simulink model "Model_HVAC_final_Lidia Garcia"  (R2020b)
settings: Solver=VariableStepAuto  StartTime=0.0  StopTime=8760  RelTol=1e-3
undefined symbols (not defined in the file or in its folder): sigbuilder_block
settings Model: Creator=HP  LastModifiedBy=HP
settings SolverCC: ZeroCrossAlgorithm=Adaptive
settings DebuggingCC: IgnoredZcDiagnostic=none  ArithmeticOperatorsInVariantConditions=warning
settings SFSimCC: CustomCodeUndefinedFunction=UseInterfaceOnly

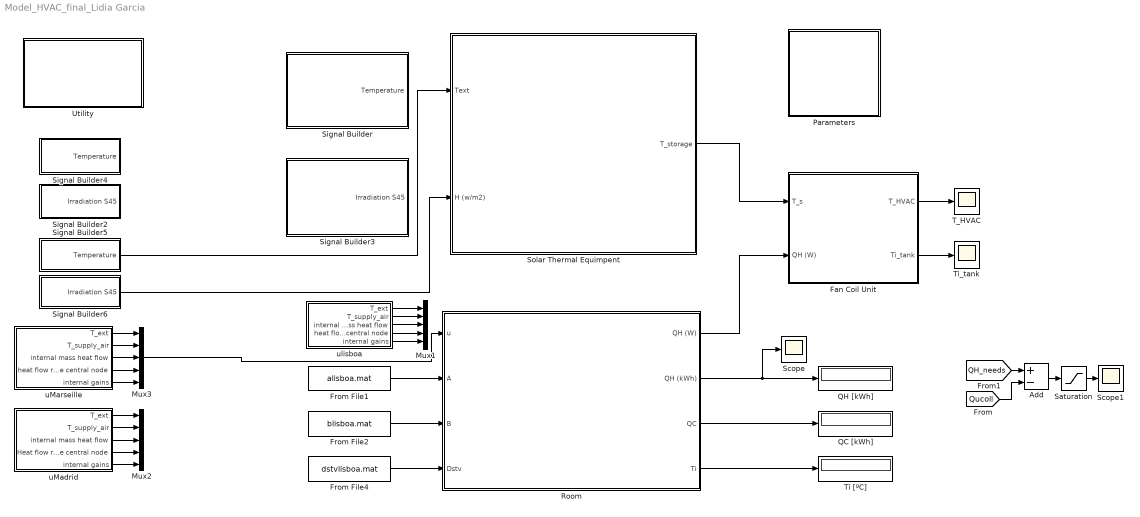
== system Model_HVAC_final_Lidia Garcia ==
  Add : Sum  Inputs=+-
  Fan Coil Unit : Subsystem
      mask Display: image('C:\Users\HP\Desktop\FCU2.jpg'); % Use "Edit Image" on toolstrip to change.
  From File1 : FromFile  FileName=alisboa.mat  SampleTime=1
  From File2 : FromFile  FileName=blisboa.mat  SampleTime=1
  From File4 : FromFile  FileName=dstvlisboa.mat  SampleTime=1
  Mux1 : Mux  Inputs=5
  Mux2 : Mux  Inputs=5
  Mux3 : Mux  Inputs=5
  Parameters : Subsystem  mask{Gamma=0, Rho=0.2, Lat=38.74, Beta=45, Eta0=0.959, a1=8.91, a2=0.047, Nc=2, Aap=4, m_brine=0.010, Cp_brine=3900, L=1.7, Eta_pump=0.8, Eta_el=0.95, H_pressure=50000, Pump_power=65, Rho_brine=1037, T_room=20, BU_power=2000, Rho_water=1000, Cp_water=4186, U_s=1, T_s_in=45, D_s=0.6, V_s=500, H_s=0.99, UA_s_ex=167, T_s_max=90, A_s_ex=1.8, U_s_ex=1.1, T_DHW=60, S_u=200, T_acq=15}
      mask prompts: Gamma "Azimuth (°)"; Rho "Albedo"; Lat "Latitude (°)"; Beta "Tilt (°)"; Eta0 "Optical efficiency"; a1 "First order coefficient"; a2 "Second order coefficient"; Nc "Number of collectors"; Aap "Absorber area (m2)"; m_brine "Flow rate per surface area (kg/s*m2)"; Cp_brine "Cp brine (J/kgK)"; L "Collector liquid volume (lt)"; Eta_pump "Pump efficiency"; Eta_el "Electrical efficiency"; H_pressure "Head pressure (Pa)"; Pump_power "Pump power (W)"; Rho_brine "Brine density (kg/m3)"; T_room "Room temperature (°C)"; BU_power "Back-up power (W)"; Rho_water "Water density (kg/m3)"; Cp_water "Cp water (J/kgK)"; U_s "Storage U (W/m2K)"; T_s_in "Initial storage temperature (°C)"; D_s "Storage diameter (m)"; V_s "Storage volume (lt)"; H_s "Storage height (m)"; UA_s_ex "Solar exchanger UA (W/K)"; T_s_max "Maximum storage temperature (°C)"; A_s_ex "Heat exchanger area (m2)"; U_s_ex "U-value heat exchanger (W/m2K)"; T_DHW "DHW temperature (°C)"; S_u "Building energetic surface (m2)"; T_acq "Aqueduct temperature (°C)"
      mask Display: image(imread('images.jpg'))
  QC [kWh] : Display
      settings: Format=bank  SampleTime=1
  QH [kWh] : Display
      settings: Format=bank  SampleTime=1
  Room : Subsystem
      mask Display: image('roomoffice.jpg'); % Use "Edit Image" on toolstrip to change.
  Saturation : Saturate  UpperLimit=5000  LowerLimit=0
  Scope : Scope
  Scope1 : Scope
  Signal Builder : Subsystem  Tag=STV Subsys  LoadFcn=sigbuilder_block('load');  StartFcn=sigbuilder_block('start');  StopFcn=sigbuilder_block('stop');  ClipboardFcn=sigbuilder_block('clipboard');  mask(Sigbuilder block){tuvar=[0:10]}
      mask help: Simulink:masks:SigbuilderBlock_MD
      mask init:
      | if ~strcmp(get_param(bdroot(gcbh),'SimulationStatus'),'stopped') tuvar = sigbuilder_block('maskInit'); end
      settings: CopyFcn=sigbuilder_block('copy');  DeleteFcn=sigbuilder_block('delete');  ModelCloseFcn=sigbuilder_block('modelClose');  PreSaveFcn=sigbuilder_block('preSave');  PauseFcn=sigbuilder_block('pause');  ContinueFcn=sigbuilder_block('continue');  NameChangeFcn=sigbuilder_block('namechange');  OpenFcn=sigbuilder_block('open',[437.6 153 550.4 359.25 ]);  CloseFcn=sigbuilder_block('close');
      mask Display: plot(0, 0, 100, 100,[2, 2, 32, 32, 2], [68, 8, 8, 68, 68],[32, 2], [38, 38], [32, 19, 2],[53, 60, 44], [32, 17, 17, 2],[16, 16, 31, 31]);txt = getActiveGroup(gcbh);text(2, 100, txt,'verticalAlignment', 'top');
  Signal Builder2 : Subsystem  Tag=STV Subsys  LoadFcn=sigbuilder_block('load');  StartFcn=sigbuilder_block('start');  StopFcn=sigbuilder_block('stop');  ClipboardFcn=sigbuilder_block('clipboard');  mask(Sigbuilder block){tuvar=[0:10]}
      mask help: Simulink:masks:SigbuilderBlock_MD
      mask init:
      | if ~strcmp(get_param(bdroot(gcbh),'SimulationStatus'),'stopped') tuvar = sigbuilder_block('maskInit'); end
      settings: CopyFcn=sigbuilder_block('copy');  DeleteFcn=sigbuilder_block('delete');  ModelCloseFcn=sigbuilder_block('modelClose');  PreSaveFcn=sigbuilder_block('preSave');  PauseFcn=sigbuilder_block('pause');  ContinueFcn=sigbuilder_block('continue');  NameChangeFcn=sigbuilder_block('namechange');  OpenFcn=sigbuilder_block('open',[437.6 153 550.4 359.25 ]);  CloseFcn=sigbuilder_block('close');
      mask Display: plot(0, 0, 100, 100,[2, 2, 32, 32, 2], [68, 8, 8, 68, 68],[32, 2], [38, 38], [32, 19, 2],[53, 60, 44], [32, 17, 17, 2],[16, 16, 31, 31]);txt = getActiveGroup(gcbh);text(2, 100, txt,'verticalAlignment', 'top');
  Signal Builder3 : Subsystem  Tag=STV Subsys  LoadFcn=sigbuilder_block('load');  StartFcn=sigbuilder_block('start');  StopFcn=sigbuilder_block('stop');  ClipboardFcn=sigbuilder_block('clipboard');  mask(Sigbuilder block){tuvar=[0:10]}
      mask help: Simulink:masks:SigbuilderBlock_MD
      mask init:
      | if ~strcmp(get_param(bdroot(gcbh),'SimulationStatus'),'stopped') tuvar = sigbuilder_block('maskInit'); end
      settings: CopyFcn=sigbuilder_block('copy');  DeleteFcn=sigbuilder_block('delete');  ModelCloseFcn=sigbuilder_block('modelClose');  PreSaveFcn=sigbuilder_block('preSave');  PauseFcn=sigbuilder_block('pause');  ContinueFcn=sigbuilder_block('continue');  NameChangeFcn=sigbuilder_block('namechange');  OpenFcn=sigbuilder_block('open',[437.6 153 550.4 359.25 ]);  CloseFcn=sigbuilder_block('close');
      mask Display: plot(0, 0, 100, 100,[2, 2, 32, 32, 2], [68, 8, 8, 68, 68],[32, 2], [38, 38], [32, 19, 2],[53, 60, 44], [32, 17, 17, 2],[16, 16, 31, 31]);txt = getActiveGroup(gcbh);text(2, 100, txt,'verticalAlignment', 'top');
  Signal Builder4 : Subsystem  Tag=STV Subsys  LoadFcn=sigbuilder_block('load');  StartFcn=sigbuilder_block('start');  StopFcn=sigbuilder_block('stop');  ClipboardFcn=sigbuilder_block('clipboard');  mask(Sigbuilder block){tuvar=[0:10]}
      mask help: Simulink:masks:SigbuilderBlock_MD
      mask init:
      | if ~strcmp(get_param(bdroot(gcbh),'SimulationStatus'),'stopped') tuvar = sigbuilder_block('maskInit'); end
      settings: CopyFcn=sigbuilder_block('copy');  DeleteFcn=sigbuilder_block('delete');  ModelCloseFcn=sigbuilder_block('modelClose');  PreSaveFcn=sigbuilder_block('preSave');  PauseFcn=sigbuilder_block('pause');  ContinueFcn=sigbuilder_block('continue');  NameChangeFcn=sigbuilder_block('namechange');  OpenFcn=sigbuilder_block('open',[437.6 153 550.4 359.25 ]);  CloseFcn=sigbuilder_block('close');
      mask Display: plot(0, 0, 100, 100,[2, 2, 32, 32, 2], [68, 8, 8, 68, 68],[32, 2], [38, 38], [32, 19, 2],[53, 60, 44], [32, 17, 17, 2],[16, 16, 31, 31]);txt = getActiveGroup(gcbh);text(2, 100, txt,'verticalAlignment', 'top');
  Signal Builder5 : Subsystem  Tag=STV Subsys  LoadFcn=sigbuilder_block('load');  StartFcn=sigbuilder_block('start');  StopFcn=sigbuilder_block('stop');  ClipboardFcn=sigbuilder_block('clipboard');  mask(Sigbuilder block){tuvar=[0:10]}
      mask help: Simulink:masks:SigbuilderBlock_MD
      mask init:
      | if ~strcmp(get_param(bdroot(gcbh),'SimulationStatus'),'stopped') tuvar = sigbuilder_block('maskInit'); end
      settings: CopyFcn=sigbuilder_block('copy');  DeleteFcn=sigbuilder_block('delete');  ModelCloseFcn=sigbuilder_block('modelClose');  PreSaveFcn=sigbuilder_block('preSave');  PauseFcn=sigbuilder_block('pause');  ContinueFcn=sigbuilder_block('continue');  NameChangeFcn=sigbuilder_block('namechange');  OpenFcn=sigbuilder_block('open',[437.6 153 550.4 359.25 ]);  CloseFcn=sigbuilder_block('close');
      mask Display: plot(0, 0, 100, 100,[2, 2, 32, 32, 2], [68, 8, 8, 68, 68],[32, 2], [38, 38], [32, 19, 2],[53, 60, 44], [32, 17, 17, 2],[16, 16, 31, 31]);txt = getActiveGroup(gcbh);text(2, 100, txt,'verticalAlignment', 'top');
  Signal Builder6 : Subsystem  Tag=STV Subsys  LoadFcn=sigbuilder_block('load');  StartFcn=sigbuilder_block('start');  StopFcn=sigbuilder_block('stop');  ClipboardFcn=sigbuilder_block('clipboard');  mask(Sigbuilder block){tuvar=[0:10]}
      mask help: Simulink:masks:SigbuilderBlock_MD
      mask init:
      | if ~strcmp(get_param(bdroot(gcbh),'SimulationStatus'),'stopped') tuvar = sigbuilder_block('maskInit'); end
      settings: CopyFcn=sigbuilder_block('copy');  DeleteFcn=sigbuilder_block('delete');  ModelCloseFcn=sigbuilder_block('modelClose');  PreSaveFcn=sigbuilder_block('preSave');  PauseFcn=sigbuilder_block('pause');  ContinueFcn=sigbuilder_block('continue');  NameChangeFcn=sigbuilder_block('namechange');  OpenFcn=sigbuilder_block('open',[440.25 156.75 544.5 355.5 ]);  CloseFcn=sigbuilder_block('close');
      mask Display: plot(0, 0, 100, 100,[2, 2, 32, 32, 2], [68, 8, 8, 68, 68],[32, 2], [38, 38], [32, 19, 2],[53, 60, 44], [32, 17, 17, 2],[16, 16, 31, 31]);txt = getActiveGroup(gcbh);text(2, 100, txt,'verticalAlignment', 'top');
  Solar Thermal Equimpent : Subsystem
      mask Display: image('C:\Users\HP\Desktop\ST2.jpg'); % Use "Edit Image" on toolstrip to change.
  T_HVAC : Scope
  Ti [ºC] : Display
      settings: Format=bank  SampleTime=1
  Ti_tank : Scope
  Utility : Subsystem
  uMadrid : Subsystem  Tag=STV Subsys  LoadFcn=sigbuilder_block('load');  StartFcn=sigbuilder_block('start');  StopFcn=sigbuilder_block('stop');  ClipboardFcn=sigbuilder_block('clipboard');  mask(Sigbuilder block){tuvar=[0:10]}
      mask help: Simulink:masks:SigbuilderBlock_MD
      mask init:
      | if ~strcmp(get_param(bdroot(gcbh),'SimulationStatus'),'stopped') tuvar = sigbuilder_block('maskInit'); end
      settings: CopyFcn=sigbuilder_block('copy');  DeleteFcn=sigbuilder_block('delete');  ModelCloseFcn=sigbuilder_block('modelClose');  PreSaveFcn=sigbuilder_block('preSave');  PauseFcn=sigbuilder_block('pause');  ContinueFcn=sigbuilder_block('continue');  NameChangeFcn=sigbuilder_block('namechange');  OpenFcn=sigbuilder_block('open',[437.6 153 550.4 359.25 ]);  CloseFcn=sigbuilder_block('close');
      mask Display: plot(0, 0, 100, 100,[2, 2, 32, 32, 2], [68, 8, 8, 68, 68],[32, 2], [38, 38], [32, 19, 2],[53, 60, 44], [32, 17, 17, 2],[16, 16, 31, 31]);txt = getActiveGroup(gcbh);text(2, 100, txt,'verticalAlignment', 'top');
  uMarseille : Subsystem  Tag=STV Subsys  LoadFcn=sigbuilder_block('load');  StartFcn=sigbuilder_block('start');  StopFcn=sigbuilder_block('stop');  ClipboardFcn=sigbuilder_block('clipboard');  mask(Sigbuilder block){tuvar=[0:10]}
      mask help: Simulink:masks:SigbuilderBlock_MD
      mask init:
      | if ~strcmp(get_param(bdroot(gcbh),'SimulationStatus'),'stopped') tuvar = sigbuilder_block('maskInit'); end
      settings: CopyFcn=sigbuilder_block('copy');  DeleteFcn=sigbuilder_block('delete');  ModelCloseFcn=sigbuilder_block('modelClose');  PreSaveFcn=sigbuilder_block('preSave');  PauseFcn=sigbuilder_block('pause');  ContinueFcn=sigbuilder_block('continue');  NameChangeFcn=sigbuilder_block('namechange');  OpenFcn=sigbuilder_block('open',[437.6 153 550.4 359.25 ]);  CloseFcn=sigbuilder_block('close');
      mask Display: plot(0, 0, 100, 100,[2, 2, 32, 32, 2], [68, 8, 8, 68, 68],[32, 2], [38, 38], [32, 19, 2],[53, 60, 44], [32, 17, 17, 2],[16, 16, 31, 31]);txt = getActiveGroup(gcbh);text(2, 100, txt,'verticalAlignment', 'top');
  ulisboa : Subsystem  Tag=STV Subsys  LoadFcn=sigbuilder_block('load');  StartFcn=sigbuilder_block('start');  StopFcn=sigbuilder_block('stop');  ClipboardFcn=sigbuilder_block('clipboard');  mask(Sigbuilder block){tuvar=[0:10]}
      mask help: Simulink:masks:SigbuilderBlock_MD
      mask init:
      | if ~strcmp(get_param(bdroot(gcbh),'SimulationStatus'),'stopped') tuvar = sigbuilder_block('maskInit'); end
      settings: CopyFcn=sigbuilder_block('copy');  DeleteFcn=sigbuilder_block('delete');  ModelCloseFcn=sigbuilder_block('modelClose');  PreSaveFcn=sigbuilder_block('preSave');  PauseFcn=sigbuilder_block('pause');  ContinueFcn=sigbuilder_block('continue');  NameChangeFcn=sigbuilder_block('namechange');  OpenFcn=sigbuilder_block('open',[6 30 1012.5 447.75 ]);  CloseFcn=sigbuilder_block('close');
      mask Display: plot(0, 0, 100, 100,[2, 2, 32, 32, 2], [68, 8, 8, 68, 68],[32, 2], [38, 38], [32, 19, 2],[53, 60, 44], [32, 17, 17, 2],[16, 16, 31, 31]);txt = getActiveGroup(gcbh);text(2, 100, txt,'verticalAlignment', 'top');
  wires:
  Room/4(Ti) -> Ti [ºC]/1
  From File4/1 -> Room/4(Dstv)
  Room/2(QH (kWh)) -> Scope/1, QH [kWh]/1
  From File1/1 -> Room/2(A)
  From File2/1 -> Room/3(B)
  Room/3(QC) -> QC [kWh]/1
  ulisboa/3(internal mass heat flow) -> Mux1/3
  ulisboa/4(heat flow rate to the central node) -> Mux1/4
  ulisboa/5(internal gains) -> Mux1/5
  ulisboa/1(T_ext) -> Mux1/1
  uMadrid/2(T_supply_air) -> Mux2/2
  uMadrid/4(Heat flow rate to the central node) -> Mux2/4
  uMadrid/1(T_ext) -> Mux2/1
  uMadrid/3(internal mass heat flow) -> Mux2/3
  uMadrid/5(internal gains) -> Mux2/5
  uMarseille/4(heat flow rate to the central node) -> Mux3/4
  uMarseille/1(T_ext) -> Mux3/1
  uMarseille/3(internal mass heat flow) -> Mux3/3
  uMarseille/5(internal gains) -> Mux3/5
  uMarseille/2(T_supply_air) -> Mux3/2
  ulisboa/2(T_supply_air) -> Mux1/2
  Room/1(QH (W)) -> Fan Coil Unit/2(QH (W))
  Fan Coil Unit/1(T_HVAC) -> T_HVAC/1
  Fan Coil Unit/2(Ti_tank) -> Ti_tank/1
  Solar Thermal Equimpent/1(T_storage) -> Fan Coil Unit/1(T_s)
  [QH_needs] -> Add/1
  [Qucoll] -> Add/2
  Add/1 -> Saturation/1
  Saturation/1 -> Scope1/1
  Mux3/1 -> Room/1(u)
  Signal Builder6/1(Irradiation S45) -> Solar Thermal Equimpent/2(H (w/m2))
  Signal Builder5/1(Temperature) -> Solar Thermal Equimpent/1(Text)

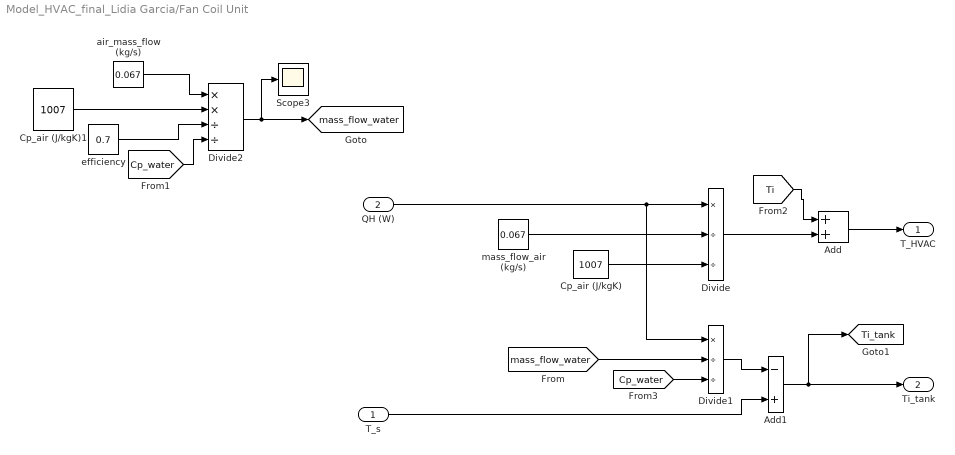
== system Model_HVAC_final_Lidia Garcia/Fan Coil Unit ==
  T_s : Inport
  QH (W) : Inport  Port=2
  Add : Sum
  Add1 : Sum  Inputs=-+
  Cp_air (J/kgK) : Constant  Value=1007  SampleTime=-1
  Cp_air (J/kgK)1 : Constant  Value=1007  SampleTime=-1
  Divide : Product  Inputs=*//
  Divide1 : Product  Inputs=*//
  Divide2 : Product  Inputs=**//
  Scope3 : Scope
  air_mass_flow (kg/s) : Constant  Value=0.067  SampleTime=-1
  efficiency : Constant  Value=0.7  SampleTime=-1
  mass_flow_air (kg/s) : Constant  Value=0.067  SampleTime=-1
  T_HVAC : Outport
  Ti_tank : Outport  Port=2
  tag scope: Ti_tank=global, mass_flow_water=global
  wires:
  T_s/1 -> Add1/2
  [mass_flow_water] -> Divide1/2
  [Cp_water] -> Divide1/3
  Divide1/1 -> Add1/1
  Add1/1 -> [Ti_tank], Ti_tank/1
  mass_flow_air (kg/s)/1 -> Divide/2
  Cp_air (J/kgK)/1 -> Divide/3
  QH (W)/1 -> Divide/1, Divide1/1
  Divide2/1 -> [mass_flow_water], Scope3/1
  Cp_air (J/kgK)1/1 -> Divide2/2
  air_mass_flow (kg/s)/1 -> Divide2/1
  [Cp_water] -> Divide2/4
  efficiency/1 -> Divide2/3
  Divide/1 -> Add/2
  Add/1 -> T_HVAC/1
  [Ti] -> Add/1

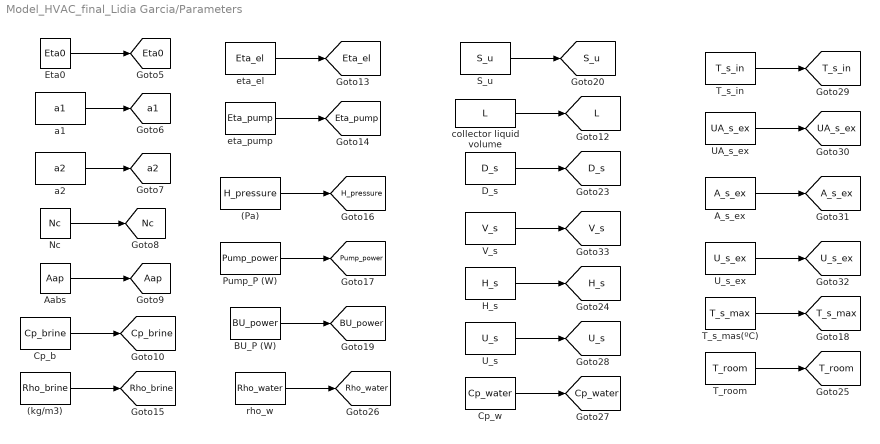
== system Model_HVAC_final_Lidia Garcia/Parameters ==
  (Pa) : Constant  Value=H_pressure  SampleTime=-1
  (kg/m3) : Constant  Value=Rho_brine  SampleTime=-1
  A_s_ex : Constant  Value=A_s_ex  SampleTime=-1
  Aabs : Constant  Value=Aap  SampleTime=-1
  BU_P (W) : Constant  Value=BU_power  SampleTime=-1
  Cp_b : Constant  Value=Cp_brine  SampleTime=-1
  Cp_w : Constant  Value=Cp_water  SampleTime=-1
  D_s : Constant  Value=D_s  SampleTime=-1
  Eta0 : Constant  Value=Eta0  SampleTime=-1
  H_s : Constant  Value=H_s  SampleTime=-1
  Nc : Constant  Value=Nc  SampleTime=-1
  Pump_P (W) : Constant  Value=Pump_power  SampleTime=-1
  S_u : Constant  Value=S_u  SampleTime=-1
  T_room : Constant  Value=T_room  SampleTime=-1
  T_s_in : Constant  Value=T_s_in  SampleTime=-1
  T_s_mas(ºC) : Constant  Value=T_s_max  SampleTime=-1
  UA_s_ex : Constant  Value=UA_s_ex  SampleTime=-1
  U_s : Constant  Value=U_s  SampleTime=-1
  U_s_ex : Constant  Value=U_s_ex  SampleTime=-1
  V_s : Constant  Value=V_s  SampleTime=-1
  a1 : Constant  Value=a1  SampleTime=-1
  a2 : Constant  Value=a2  SampleTime=-1
  collector liquid volume : Constant  Value=L  SampleTime=-1
  eta_el : Constant  Value=Eta_el  SampleTime=-1
  eta_pump : Constant  Value=Eta_pump  SampleTime=-1
  rho_w : Constant  Value=Rho_water  SampleTime=-1
  tag scope: A_s_ex=global, Aap=global, BU_power=global, Cp_brine=global, Cp_water=global, D_s=global, Eta0=global, Eta_el=global, Eta_pump=global, H_pressure=global, H_s=global, L=global, Nc=global, Pump_power=global, Rho_brine=global, Rho_water=global, S_u=global, T_room=global, T_s_in=global, T_s_max=global, UA_s_ex=global, U_s=global, U_s_ex=global, V_s=global, a1=global, a2=global
  wires:
  T_s_mas(ºC)/1 -> [T_s_max]
  Cp_w/1 -> [Cp_water]
  U_s_ex/1 -> [U_s_ex]
  rho_w/1 -> [Rho_water]
  U_s/1 -> [U_s]
  D_s/1 -> [D_s]
  V_s/1 -> [V_s]
  UA_s_ex/1 -> [UA_s_ex]
  Aabs/1 -> [Aap]
  T_room/1 -> [T_room]
  A_s_ex/1 -> [A_s_ex]
  Nc/1 -> [Nc]
  a1/1 -> [a1]
  Pump_P (W)/1 -> [Pump_power]
  (Pa)/1 -> [H_pressure]
  T_s_in/1 -> [T_s_in]
  BU_P (W)/1 -> [BU_power]
  (kg/m3)/1 -> [Rho_brine]
  eta_pump/1 -> [Eta_pump]
  Eta0/1 -> [Eta0]
  collector liquid volume/1 -> [L]
  S_u/1 -> [S_u]
  eta_el/1 -> [Eta_el]
  Cp_b/1 -> [Cp_brine]
  a2/1 -> [a2]
  H_s/1 -> [H_s]

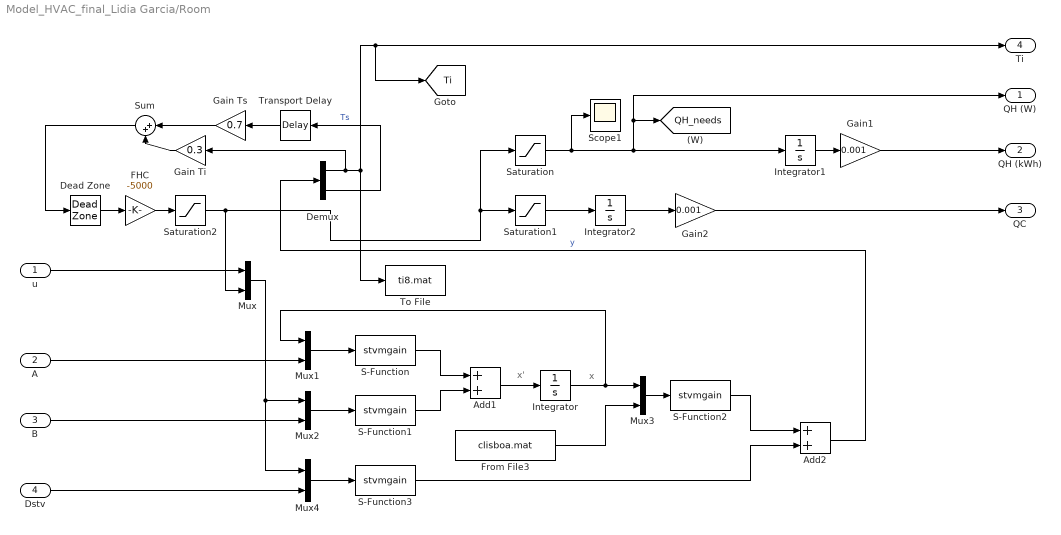
== system Model_HVAC_final_Lidia Garcia/Room ==
  note: x'
  note: x
  u : Inport
  A : Inport  Port=2
  B : Inport  Port=3
  Dstv : Inport  Port=4
  Add1 : Sum
  Add2 : Sum
  Dead Zone : DeadZone  LowerValue=20  UpperValue=26  ZeroCross=off  SaturateOnIntegerOverflow=on
  Demux : Demux  Outputs=2
  FHC : Gain  Gain=-5000
  From File3 : FromFile  FileName=clisboa.mat  SampleTime=1
  Gain Ti : Gain  Gain=0.3
  Gain Ts : Gain  Gain=0.7
  Gain1 : Gain  Gain=0.001  SampleTime=1
  Gain2 : Gain  Gain=0.001  SampleTime=1
  Integrator : Integrator  InitialCondition=18
  Integrator1 : Integrator
  Integrator2 : Integrator
  Mux : Mux  Inputs=2
  Mux1 : Mux  Inputs=[1 1]
  Mux2 : Mux  Inputs=[6 6]
  Mux3 : Mux  Inputs=[1 2]
  Mux4 : Mux  Inputs=[6 12]
  S-Function : S-Function  FunctionName=stvmgain  Parameters=1, -1  SFunctionDeploymentMode=off  EnableBusSupport=off
  S-Function1 : S-Function  FunctionName=stvmgain  Parameters=[1 1 1 1 1 1], -1  SFunctionDeploymentMode=off  EnableBusSupport=off
  S-Function2 : S-Function  FunctionName=stvmgain  Parameters=[1 ;1] -1  SFunctionDeploymentMode=off  EnableBusSupport=off
  S-Function3 : S-Function  FunctionName=stvmgain  Parameters=[1 1 1 1 1 1; 1 1 1 1 1 1], -1  SFunctionDeploymentMode=off  EnableBusSupport=off
  Saturation : Saturate  UpperLimit=20000  LowerLimit=0  SampleTime=1
  Saturation1 : Saturate  UpperLimit=0  LowerLimit=-20000  SampleTime=1
  Saturation2 : Saturate  UpperLimit=10000  LowerLimit=-10000
  Scope1 : Scope
  Sum : Sum  Inputs=|++
  To File : ToFile  Filename=ti8.mat  SampleTime=1
  Transport Delay : TransportDelay
  QH (W) : Outport
  QH (kWh) : Outport  Port=2  VectorParamsAs1DForOutWhenUnconnected=off
  QC : Outport  Port=3  VectorParamsAs1DForOutWhenUnconnected=off
  Ti : Outport  Port=4  VectorParamsAs1DForOutWhenUnconnected=off
  tag scope: QH_needs=global, Ti=global
  wires:
  Sum/1 -> Dead Zone/1
  Mux3/1 -> S-Function2/1
  Demux/1 -> Gain Ti/1, [Ti], Ti/1, To File/1
  Mux2/1 -> S-Function1/1
  Saturation2/1 -> Mux/2, Saturation1/1, Saturation/1
  Mux/1 -> Mux2/1, Mux4/1
  Saturation/1 -> Scope1/1, Integrator1/1, [QH_needs], QH (W)/1
  Gain1/1 -> QH (kWh)/1
  S-Function/1 -> Add1/1
  Mux4/1 -> S-Function3/1
  Integrator/1 -> Mux3/1, Mux1/1
  FHC/1 -> Saturation2/1
  Saturation1/1 -> Integrator2/1
  Gain Ts/1 -> Sum/1
  Mux1/1 -> S-Function/1
  S-Function3/1 -> Add2/2
  Transport Delay/1 -> Gain Ts/1
  Dead Zone/1 -> FHC/1
  Gain Ti/1 -> Sum/2
  S-Function1/1 -> Add1/2
  Integrator2/1 -> Gain2/1
  Demux/2 -> Transport Delay/1  "Ts"
  B/1 -> Mux2/2
  Add1/1 -> Integrator/1
  Gain2/1 -> QC/1
  From File3/1 -> Mux3/2
  A/1 -> Mux1/2
  S-Function2/1 -> Add2/1
  Integrator1/1 -> Gain1/1
  Add2/1 -> Demux/1  "y"
  Dstv/1 -> Mux4/2
  u/1 -> Mux/1

== system Model_HVAC_final_Lidia Garcia/Signal Builder ==
  Demux : Demux  Tag=STV Demux  Outputs=1
      settings: DisplayOption=none
  FromWs : FromWorkspace  Tag=STV FromWs  VariableName=tuvar
      SigBuilderData=|
      | common.afterFinalStr = 'Extrapolate'
      | common.sampleTime = 0
      | dataSet.timeRange = [0 8760]
      | dataSet.name = 'Lisbon'
      | sbobj.Groups.Name = 'Lisbon'
      | sbobj.Groups.Signals.Name = 'Temperature'
      | sbobj.Groups.Signals.XData = [0 1 2 3 4 5 6 7 8 9 10 11 ... (8761 elements, 1x8761)]
      | sbobj.Groups.Signals.YData = [10.3 10.3 10.5 10.4 10.4 10.3 10.2 10.1 10 10.2 10.7 11.6 ... (8761 elements, 1x8761)]
      | sbobj.Groups.TimeRange = [0 8760]
  Temperature : Outport  Tag=STV Outport
  wires:
  FromWs/1 -> Demux/1
  Demux/1 -> Temperature/1

== system Model_HVAC_final_Lidia Garcia/Signal Builder2 ==
  Demux : Demux  Tag=STV Demux  Outputs=1
      settings: DisplayOption=none
  FromWs : FromWorkspace  Tag=STV FromWs  VariableName=tuvar
      SigBuilderData=|
      | common.afterFinalStr = 'Extrapolate'
      | common.sampleTime = 0
      | dataSet.timeRange = [0 8760]
      | dataSet.name = 'Madrid'
      | sbobj.Groups.Name = 'Madrid'
      | sbobj.Groups.Signals.Name = 'Irradiation S45'
      | sbobj.Groups.Signals.XData = [0 2 3 4 5 6 7 8 9 10 11 12 ... (8760 elements, 1x8760)]
      | sbobj.Groups.Signals.YData = [0 0 0 0 0 0 0 0 1.76568542495 17.6568542495 95.9744879539 148.273951851 ... (8760 elements, 1x8760)]
      | sbobj.Groups.TimeRange = [0 8760]
  Irradiation S45 : Outport  Tag=STV Outport
  wires:
  FromWs/1 -> Demux/1
  Demux/1 -> Irradiation S45/1

== system Model_HVAC_final_Lidia Garcia/Signal Builder3 ==
  Demux : Demux  Tag=STV Demux  Outputs=1
      settings: DisplayOption=none
  FromWs : FromWorkspace  Tag=STV FromWs  VariableName=tuvar
      SigBuilderData=|
      | common.afterFinalStr = 'Extrapolate'
      | common.sampleTime = 0
      | dataSet.timeRange = [0 8760]
      | dataSet.name = 'Lisbon'
      | sbobj.Groups.Name = 'Lisbon'
      | sbobj.Groups.Signals.Name = 'Irradiation S45'
      | sbobj.Groups.Signals.XData = [0 2 3 4 5 6 7 8 9 10 11 12 ... (8759 elements, 1x8759)]
      | sbobj.Groups.Signals.YData = [0 0 0 0 0 0 0 37.162504834 51.5011301066 101.550573461 150.372893262 151.238870404 ... (8759 elements, 1x8759)]
      | sbobj.Groups.TimeRange = [0 8760]
  Irradiation S45 : Outport  Tag=STV Outport
  wires:
  FromWs/1 -> Demux/1
  Demux/1 -> Irradiation S45/1

== system Model_HVAC_final_Lidia Garcia/Signal Builder4 ==
  Demux : Demux  Tag=STV Demux  Outputs=1
      settings: DisplayOption=none
  FromWs : FromWorkspace  Tag=STV FromWs  VariableName=tuvar
      SigBuilderData=|
      | common.afterFinalStr = 'Extrapolate'
      | common.sampleTime = 0
      | dataSet.timeRange = [0 8760]
      | dataSet.name = 'Madrid'
      | sbobj.Groups.Name = 'Madrid'
      | sbobj.Groups.Signals.Name = 'Temperature'
      | sbobj.Groups.Signals.XData = [0 2 3 4 5 6 7 8 9 10 11 12 ... (8759 elements, 1x8759)]
      | sbobj.Groups.Signals.YData = [4.4 4.4 4.4 3.9 3.9 3.3 3.3 2.8 3.3 3.9 5 6.1 ... (8759 elements, 1x8759)]
      | sbobj.Groups.TimeRange = [0 8760]
  Temperature : Outport  Tag=STV Outport
  wires:
  FromWs/1 -> Demux/1
  Demux/1 -> Temperature/1

== system Model_HVAC_final_Lidia Garcia/Signal Builder5 ==
  Demux : Demux  Tag=STV Demux  Outputs=1
      settings: DisplayOption=none
  FromWs : FromWorkspace  Tag=STV FromWs  VariableName=tuvar
      SigBuilderData=|
      | common.afterFinalStr = 'Extrapolate'
      | common.sampleTime = 0
      | dataSet.timeRange = [0 8760]
      | dataSet.name = 'Marseille'
      | sbobj.Groups.Name = 'Marseille'
      | sbobj.Groups.Signals.Name = 'Temperature'
      | sbobj.Groups.Signals.XData = [0 1 2 3 4 5 6 7 8 9 10 11 ... (8761 elements, 1x8761)]
      | sbobj.Groups.Signals.YData = [9.4 9.4 8.9 8.6 8.4 8.3 8.1 6.9 5 6 6.3 7 ... (8761 elements, 1x8761)]
      | sbobj.Groups.TimeRange = [0 8760]
  Temperature : Outport  Tag=STV Outport
  wires:
  FromWs/1 -> Demux/1
  Demux/1 -> Temperature/1

== system Model_HVAC_final_Lidia Garcia/Signal Builder6 ==
  Demux : Demux  Tag=STV Demux  Outputs=1
      settings: DisplayOption=none
  FromWs : FromWorkspace  Tag=STV FromWs  VariableName=tuvar
      SigBuilderData=|
      | common.afterFinalStr = 'Extrapolate'
      | common.sampleTime = 0
      | dataSet.timeRange = [0 8760]
      | dataSet.name = 'Marseille'
      | sbobj.Groups.Name = 'Marseille'
      | sbobj.Groups.Signals.Name = 'Irradiation S45'
      | sbobj.Groups.Signals.XData = [0 2 3 4 5 6 7 8 9 10 11 12 ... (8760 elements, 1x8760)]
      | sbobj.Groups.Signals.YData = [0 0 0 0 0 0 0 0 6.17989898732 47.6735064736 106.25422387 126.258650915 ... (8760 elements, 1x8760)]
      | sbobj.Groups.TimeRange = [0 8760]
  Irradiation S45 : Outport  Tag=STV Outport
  wires:
  FromWs/1 -> Demux/1
  Demux/1 -> Irradiation S45/1

== system Model_HVAC_final_Lidia Garcia/Solar Thermal Equimpent ==
  Text : Inport
  H (w/m2) : Inport  Port=2
  Back-up : Subsystem
      mask Display: image(imread('caldaia.jpg'))
  Collector : Subsystem
      mask Display: image(imread('collettore.jpg'))
  Pump : Subsystem
      mask Display: image(imread('pompa.jpg'))
  Solar thermal storage : Subsystem
      mask Display: image(imread('prova.jpg'))
  T_storage : Outport
  wires:
  Collector/1(Tu,coll) -> Pump/1(Tucoll (ºC))
  Back-up/1(Qbu) -> Solar thermal storage/1(Input)
  H (w/m2)/1 -> Collector/3(H (w/m2))
  Solar thermal storage/2(T_storage) -> T_storage/1
  Text/1 -> Collector/2(Text)
  Solar thermal storage/1(Ti,coll) -> Collector/1(Ti,coll)  "Ti,coll"
  Pump/1(Tupump) -> Solar thermal storage/2(Tucoll/pump)

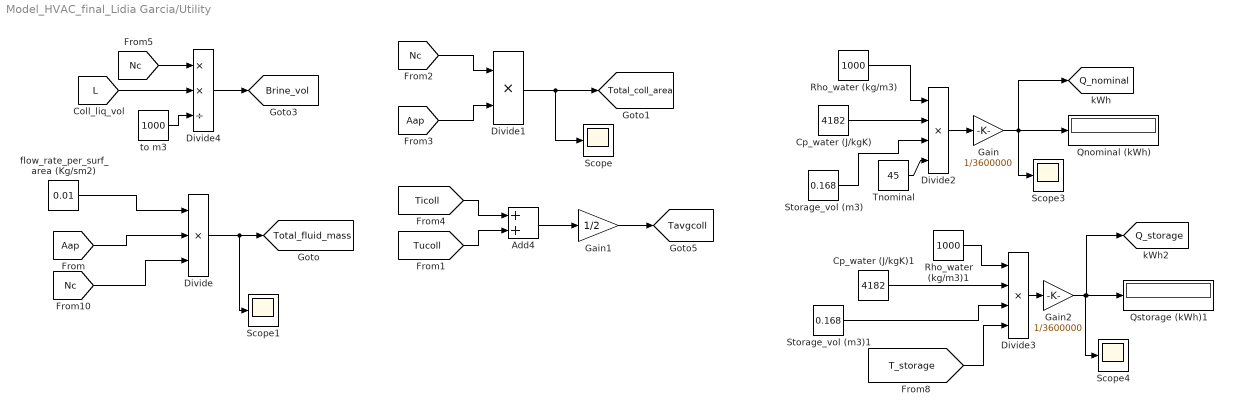
== system Model_HVAC_final_Lidia Garcia/Utility ==
  Add4 : Sum
  Cp_water (J/kgK) : Constant  Value=4182  SampleTime=-1
  Cp_water (J/kgK)1 : Constant  Value=4182  SampleTime=-1
  Divide : Product  Inputs=***
  Divide1 : Product  Inputs=**
  Divide2 : Product  Inputs=****
  Divide3 : Product  Inputs=****
  Divide4 : Product  Inputs=**/
  Gain : Gain  Gain=1/3600000
  Gain1 : Gain  Gain=1/2  SaturateOnIntegerOverflow=on  OutDataTypeStr=Inherit: Same as input  ParamDataTypeStr=Inherit: Same as input
  Gain2 : Gain  Gain=1/3600000
  Qnominal (kWh) : Display
  Qstorage (kWh)1 : Display
  Rho_water (kg/m3) : Constant  Value=1000  SampleTime=-1
  Rho_water (kg/m3)1 : Constant  Value=1000  SampleTime=-1
  Scope{,1,3..4} (4 alike) : Scope
  Storage_vol (m3) : Constant  Value=0.168  SampleTime=-1
  Storage_vol (m3)1 : Constant  Value=0.168  SampleTime=-1
  Tnominal : Constant  Value=45  SampleTime=-1
  flow_rate_per_surf_area (Kg/sm2) : Constant  Value=0.01  SampleTime=-1
  to m3 : Constant  Value=1000  SampleTime=-1
  tag scope: Brine_vol=global, Q_nominal=global, Q_storage=global, Tavgcoll=global, Total_coll_area=global, Total_fluid_mass=global
  wires:
  [Aap] -> Divide1/2
  Divide1/1 -> Scope/1, [Total_coll_area]
  [Nc] -> Divide1/1
  [Ticoll] -> Add4/1
  [Tucoll] -> Add4/2
  Add4/1 -> Gain1/1
  Gain1/1 -> [Tavgcoll]
  Cp_water (J/kgK)/1 -> Divide2/2
  Divide3/1 -> Gain2/1
  Rho_water (kg/m3)/1 -> Divide2/1
  Cp_water (J/kgK)1/1 -> Divide3/2
  Tnominal/1 -> Divide2/4
  Gain2/1 -> Qstorage (kWh)1/1, [Q_storage], Scope4/1
  [T_storage] -> Divide3/4
  Storage_vol (m3)1/1 -> Divide3/3
  Divide2/1 -> Gain/1
  Gain/1 -> [Q_nominal], Qnominal (kWh)/1, Scope3/1
  Rho_water (kg/m3)1/1 -> Divide3/1
  Storage_vol (m3)/1 -> Divide2/3
  flow_rate_per_surf_area (Kg/sm2)/1 -> Divide/1
  [Aap] -> Divide/2
  [Nc] -> Divide/3
  Divide/1 -> Scope1/1, [Total_fluid_mass]
  [Nc] -> Divide4/1
  [L] -> Divide4/2
  to m3/1 -> Divide4/3
  Divide4/1 -> [Brine_vol]

== system Model_HVAC_final_Lidia Garcia/uMadrid ==
  Demux : Demux  Tag=STV Demux  Outputs=5
      settings: DisplayOption=none
  FromWs : FromWorkspace  Tag=STV FromWs  VariableName=tuvar
      SigBuilderData=|
      | common.afterFinalStr = 'Extrapolate'
      | common.sampleTime = 0
      | dataSet.timeRange = [0 8760]
      | dataSet.name = 'Madrid'
      | sbobj.Groups.Name = 'Madrid'
      | sbobj.Groups.Signals(1).Name = 'T_ext'
      | sbobj.Groups.Signals(1).XData = [0 2 3 4 5 6 7 8 9 10 11 12 ... (8760 elements, 1x8760)]
      | sbobj.Groups.Signals(1).YData = [4.4 4.4 4.4 3.9 3.9 3.3 3.3 2.8 3.3 3.9 5 6.1 ... (8760 elements, 1x8760)]
      | sbobj.Groups.Signals(2).Name = 'T_supply_air'
      | sbobj.Groups.Signals(2).XData = [0 2 3 4 5 6 7 8 9 10 11 12 ... (8760 elements, 1x8760)]
      | sbobj.Groups.Signals(2).YData = [4.4 4.4 4.4 3.9 3.9 3.3 3.3 2.8 3.3 3.9 5 6.1 ... (8760 elements, 1x8760)]
      | sbobj.Groups.Signals(3).Name = 'internal mass heat flow'
      | sbobj.Groups.Signals(3).XData = [0 1 2 3 4 5 6 7 8 9 10 11 ... (8761 elements, 1x8761)]
      | sbobj.Groups.Signals(3).YData = [63.3950307067 63.3950307067 75.2897198881 75.0094543369 75.5336603617 75.2533948105 240.708683745 240.427180397 2000 2000 2000 2000 ... (8761 elements, 1x8761)]
      | sbobj.Groups.Signals(4).Name = 'Heat flow rate to the central node'
      | sbobj.Groups.Signals(4).XData = [0 1 2 3 4 5 6 7 8 9 10 11 ... (8761 elements, 1x8761)]
      | sbobj.Groups.Signals(4).YData = [32.2317868014 32.2317868014 38.2793757289 38.1368809719 38.4034018119 38.2609070549 122.382951616 122.239827529 -12.0329759534 -17.2014646062 281.045007622 409.965673888 ... (8761 elements, 1x8761)]
      | sbobj.Groups.Signals(5).Name = 'internal gains'
      | sbobj.Groups.Signals(5).XData = [0 2 3 4 5 6 7 8 9 10 11 12 ... (8760 elements, 1x8760)]
      | sbobj.Groups.Signals(5).YData = [150 150 150 150 150 400 400 0 0 0 0 0 ... (8760 elements, 1x8760)]
      | sbobj.Groups.TimeRange = [0 8760]
  T_ext : Outport  Tag=STV Outport
  T_supply_air : Outport  Tag=STV Outport  Port=2
  internal mass heat flow : Outport  Tag=STV Outport  Port=3
  Heat flow rate to the central node : Outport  Tag=STV Outport  Port=4
  internal gains : Outport  Tag=STV Outport  Port=5
  wires:
  FromWs/1 -> Demux/1
  Demux/1 -> T_ext/1
  Demux/2 -> T_supply_air/1
  Demux/3 -> internal mass heat flow/1
  Demux/4 -> Heat flow rate to the central node/1
  Demux/5 -> internal gains/1

== system Model_HVAC_final_Lidia Garcia/uMarseille ==
  Demux : Demux  Tag=STV Demux  Outputs=5
      settings: DisplayOption=none
  FromWs : FromWorkspace  Tag=STV FromWs  VariableName=tuvar
      SigBuilderData=|
      | common.afterFinalStr = 'Extrapolate'
      | common.sampleTime = 0
      | dataSet.timeRange = [0 8760]
      | dataSet.name = 'Marseille'
      | sbobj.Groups.Name = 'Marseille'
      | sbobj.Groups.Signals(1).Name = 'T_ext'
      | sbobj.Groups.Signals(1).XData = [0 1 2 3 4 5 6 7 8 9 10 11 ... (8761 elements, 1x8761)]
      | sbobj.Groups.Signals(1).YData = [8.9 8.9 8.6 8.4 8.3 8.1 6.9 5 6 6.3 7 9 ... (8761 elements, 1x8761)]
      | sbobj.Groups.Signals(2).Name = 'T_supply_air'
      | sbobj.Groups.Signals(2).XData = [0 1 2 3 4 5 6 7 8 9 10 11 ... (8761 elements, 1x8761)]
      | sbobj.Groups.Signals(2).YData = [8.9 8.9 8.6 8.4 8.3 8.1 6.9 5 20 20 20 20 ... (8761 elements, 1x8761)]
      | sbobj.Groups.Signals(3).Name = 'internal mass heat flow'
      | sbobj.Groups.Signals(3).XData = [0 1 2 3 4 5 6 7 8 9 10 11 ... (8761 elements, 1x8761)]
      | sbobj.Groups.Signals(3).YData = [63.3950307067 63.3950307067 75.2897198881 75.0094543369 75.5336603617 75.2533948105 240.708683745 240.427180397 2000 2000 2000 2000 ... (8761 elements, 1x8761)]
      | sbobj.Groups.Signals(4).Name = 'heat flow rate to the central node'
      | sbobj.Groups.Signals(4).XData = [0 1 2 3 4 5 6 7 8 9 10 11 ... (8761 elements, 1x8761)]
      | sbobj.Groups.Signals(4).YData = [32.2317868014 32.2317868014 38.2793757289 38.1368809719 38.4034018119 38.2609070549 122.382951616 122.239827529 -12.0329759534 -17.2014646062 281.045007622 409.965673888 ... (8761 elements, 1x8761)]
      | sbobj.Groups.Signals(5).Name = 'internal gains'
      | sbobj.Groups.Signals(5).XData = [0 2 3 4 5 6 7 8 9 10 11 12 ... (8760 elements, 1x8760)]
      | sbobj.Groups.Signals(5).YData = [150 150 150 150 150 400 400 0 0 0 0 0 ... (8760 elements, 1x8760)]
      | sbobj.Groups.TimeRange = [0 8760]
  T_ext : Outport  Tag=STV Outport
  T_supply_air : Outport  Tag=STV Outport  Port=2
  internal mass heat flow : Outport  Tag=STV Outport  Port=3
  heat flow rate to the central node : Outport  Tag=STV Outport  Port=4
  internal gains : Outport  Tag=STV Outport  Port=5
  wires:
  FromWs/1 -> Demux/1
  Demux/1 -> T_ext/1
  Demux/2 -> T_supply_air/1
  Demux/3 -> internal mass heat flow/1
  Demux/4 -> heat flow rate to the central node/1
  Demux/5 -> internal gains/1

== system Model_HVAC_final_Lidia Garcia/ulisboa ==
  Demux : Demux  Tag=STV Demux  Outputs=5
      settings: DisplayOption=none
  FromWs : FromWorkspace  Tag=STV FromWs  VariableName=tuvar
      SigBuilderData=|
      | common.afterFinalStr = 'Extrapolate'
      | common.sampleTime = 0
      | dataSet.timeRange = [0 9000]
      | dataSet.name = 'Lisbon'
      | sbobj.Groups.Name = 'Lisbon'
      | sbobj.Groups.Signals(1).Name = 'T_ext'
      | sbobj.Groups.Signals(1).XData = [0 1 2 3 4 5 6 7 8 9 10 11 ... (8762 elements, 1x8762)]
      | sbobj.Groups.Signals(1).YData = [10.3 10.3 10.5 10.4 10.4 10.3 10.2 10.1 10 10.2 10.7 11.6 ... (8762 elements, 1x8762)]
      | sbobj.Groups.Signals(2).Name = 'T_supply_air'
      | sbobj.Groups.Signals(2).XData = [0 1 2 3 4 5 6 7 8 9 10 11 ... (8762 elements, 1x8762)]
      | sbobj.Groups.Signals(2).YData = [10.3 10.3 10.5 10.4 10.4 10.3 10.2 10.1 20 20 20 20 ... (8762 elements, 1x8762)]
      | sbobj.Groups.Signals(3).Name = 'internal mass heat flow'
      | sbobj.Groups.Signals(3).XData = [0 1 2 3 4 5 6 7 8 9 10 11 ... (8762 elements, 1x8762)]
      | sbobj.Groups.Signals(3).YData = [63.3950307067 63.3950307067 75.2897198881 75.0094543369 75.5336603617 75.2533948105 240.708683745 240.427180397 2000 2000 2000 2000 ... (8762 elements, 1x8762)]
      | sbobj.Groups.Signals(4).Name = 'heat flow rate to the central node'
      | sbobj.Groups.Signals(4).XData = [0 1 2 3 4 5 6 7 8 9 10 11 ... (8762 elements, 1x8762)]
      | sbobj.Groups.Signals(4).YData = [32.2317868014 32.2317868014 38.2793757289 38.1368809719 38.4034018119 38.2609070549 122.382951616 122.239827529 -12.0329759534 -17.2014646062 281.045007622 409.965673888 ... (8762 elements, 1x8762)]
      | sbobj.Groups.Signals(5).Name = 'internal gains'
      | sbobj.Groups.Signals(5).XData = [0 2 3 4 5 6 7 8 9 10 11 12 ... (8760 elements, 1x8760)]
      | sbobj.Groups.Signals(5).YData = [150 150 150 150 150 400 400 0 0 0 0 0 ... (8760 elements, 1x8760)]
      | sbobj.Groups.TimeRange = [0 9000]
  T_ext : Outport  Tag=STV Outport
  T_supply_air : Outport  Tag=STV Outport  Port=2
  internal mass heat flow : Outport  Tag=STV Outport  Port=3
  heat flow rate to the central node : Outport  Tag=STV Outport  Port=4
  internal gains : Outport  Tag=STV Outport  Port=5
  wires:
  FromWs/1 -> Demux/1
  Demux/1 -> T_ext/1
  Demux/2 -> T_supply_air/1
  Demux/3 -> internal mass heat flow/1
  Demux/4 -> heat flow rate to the central node/1
  Demux/5 -> internal gains/1

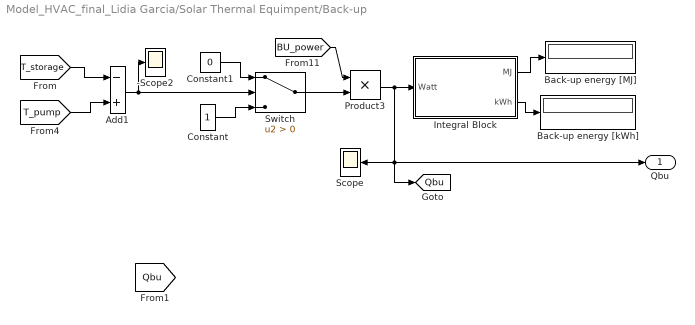
== system Model_HVAC_final_Lidia Garcia/Solar Thermal Equimpent/Back-up ==
  -Scope2 : Scope
  Add1 : Sum  Inputs=-+
  Back-up energy [MJ] : Display
  Back-up energy [kWh] : Display
  Constant : Constant  SampleTime=-1
  Constant1 : Constant  Value=0  SampleTime=-1
  Integral Block : Subsystem
  Product3 : Product  Inputs=**  SaturateOnIntegerOverflow=on  OutDataTypeStr=Inherit: Same as first input
  Scope : Scope
  Switch : Switch  Criteria=u2 > Threshold
  Qbu : Outport
  tag scope: Qbu=global
  wires:
  [T_storage] -> Add1/1
  Add1/1 -> Switch/2, -Scope2/1
  Switch/1 -> Product3/2
  Product3/1 -> Integral Block/1(Watt), Qbu/1, Scope/1, [Qbu]
  Integral Block/1(MJ) -> Back-up energy [MJ]/1
  Integral Block/2(kWh) -> Back-up energy [kWh]/1
  [T_pump] -> Add1/2
  [BU_power] -> Product3/1
  Constant1/1 -> Switch/1
  Constant/1 -> Switch/3

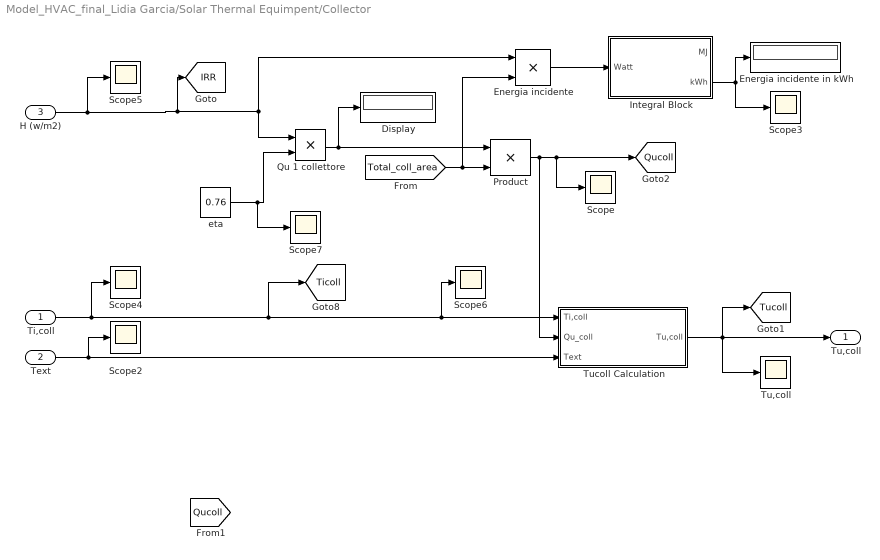
== system Model_HVAC_final_Lidia Garcia/Solar Thermal Equimpent/Collector ==
  Ti,coll : Inport
  Text : Inport  Port=2
  H (w/m2) : Inport  Port=3
  Display : Display
  Energia incidente : Product  RndMeth=Zero
  Energia incidente in kWh : Display
  Integral Block : Subsystem
  Product : Product  RndMeth=Zero
  Qu 1 collettore : Product  RndMeth=Zero
  Scope{,2..7} (7 alike) : Scope
  "Tu,coll " : Scope
  Tucoll Calculation : Subsystem
  eta : Constant  Value=0.76  SampleTime=-1
  Tu,coll : Outport
  tag scope: IRR=global, Qucoll=global, Ticoll=global, Tucoll=global
  wires:
  Qu 1 collettore/1 -> Display/1, Product/1
  Tucoll Calculation/1(Tu,coll) -> "Tu,coll "/1, [Tucoll], Tu,coll/1
  Energia incidente/1 -> Integral Block/1(Watt)
  Integral Block/2(kWh) -> Scope3/1, Energia incidente in kWh/1
  [Total_coll_area] -> Product/2, Energia incidente/2
  H (w/m2)/1 -> [IRR], Qu 1 collettore/1, Energia incidente/1, Scope5/1
  Ti,coll/1 -> Scope4/1, Tucoll Calculation/1(Ti,coll), Scope6/1, [Ticoll]
  Text/1 -> Tucoll Calculation/3(Text), Scope2/1
  eta/1 -> Scope7/1, Qu 1 collettore/2
  Product/1 -> Scope/1, [Qucoll], Tucoll Calculation/2(Qu_coll)

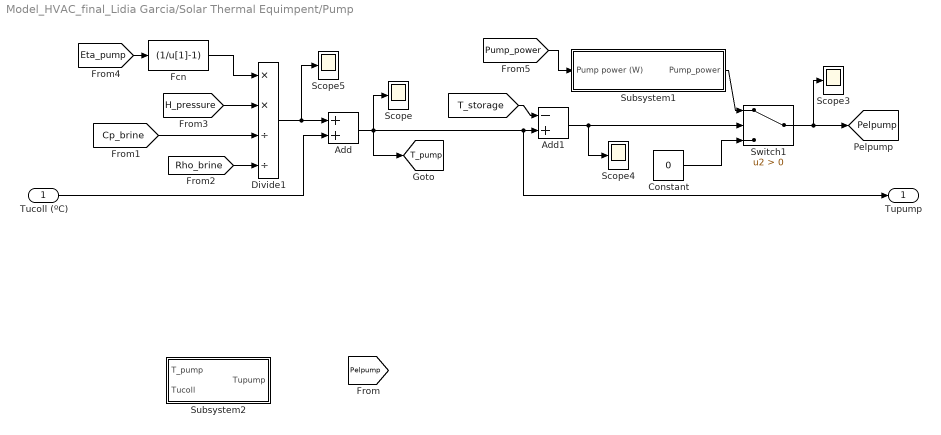
== system Model_HVAC_final_Lidia Garcia/Solar Thermal Equimpent/Pump ==
  Tucoll (ºC) : Inport
  Add : Sum
  Add1 : Sum  Inputs=-+
  Constant : Constant  Value=0
  Divide1 : Product  Inputs=**//
  Fcn : Fcn  Expr=(1/u[1]-1)
  Scope{,3..5} (4 alike) : Scope
  Subsystem1 : Subsystem
  Subsystem2 : Subsystem
  Switch1 : Switch  Criteria=u2 > Threshold
  Tupump : Outport
  tag scope: Pelpump=global, T_pump=global
  wires:
  [Eta_pump] -> Fcn/1
  Add1/1 -> Switch1/2, Scope4/1
  Subsystem1/1(Pump_power) -> Switch1/1
  Divide1/1 -> Scope5/1, Add/1
  Constant/1 -> Switch1/3
  [Rho_brine] -> Divide1/4
  [Pump_power] -> Subsystem1/1(Pump power (W))
  [H_pressure] -> Divide1/2
  Fcn/1 -> Divide1/1
  [Cp_brine] -> Divide1/3
  Switch1/1 -> [Pelpump], Scope3/1
  [T_storage] -> Add1/1
  Add/1 -> [T_pump], Tupump/1, Add1/2, Scope/1
  Tucoll (ºC)/1 -> Add/2

== system Model_HVAC_final_Lidia Garcia/Solar Thermal Equimpent/Solar thermal storage ==
  Input : Inport
  Tucoll/pump : Inport  Port=2
  Divide : Product  Inputs=*/
  Scope : Scope
  Subsystem : Subsystem
  to m3 : Constant  Value=1000  SampleTime=-1
  Ti,coll : Outport
  T_storage : Outport  Port=2
  tag scope: Qbu1=global
  wires:
  Subsystem/2(T_storage) -> T_storage/1
  to m3/1 -> Divide/2
  [V_s] -> Divide/1
  Divide/1 -> Scope/1, Subsystem/1(S_v (m3))
  Tucoll/pump/1 -> Subsystem/2(Tucoll/ppump)
  Subsystem/1(Ti,coll) -> Ti,coll/1
  Input/1 -> [Qbu1]

== system Model_HVAC_final_Lidia Garcia/Solar Thermal Equimpent/Back-up/Integral Block ==
  Watt : Inport
  Integrator : Integrator
  J to MJ : Gain  Gain=1/1000000
  MJ to kWh : Gain  Gain=1/3.6
  MJ1 : Display
  Scope1 : Scope
  Scope2 : Scope
  kWh1 : Display
  MJ : Outport  VectorParamsAs1DForOutWhenUnconnected=off
  kWh : Outport  Port=2  VectorParamsAs1DForOutWhenUnconnected=off
  wires:
  Integrator/1 -> J to MJ/1
  Watt/1 -> Integrator/1
  J to MJ/1 -> Scope1/1, MJ1/1, MJ/1, MJ to kWh/1
  MJ to kWh/1 -> Scope2/1, kWh1/1, kWh/1

== system Model_HVAC_final_Lidia Garcia/Solar Thermal Equimpent/Collector/Integral Block ==
  Watt : Inport
  J to MJ : Gain  Gain=1/1000000
  MJ to kWh : Gain  Gain=1/3.6
  MJ1 : Display
  Scope1 : Scope
  Scope2 : Scope
  kWh1 : Display
  MJ : Outport  VectorParamsAs1DForOutWhenUnconnected=off
  kWh : Outport  Port=2  VectorParamsAs1DForOutWhenUnconnected=off
  wires:
  Watt/1 -> J to MJ/1
  J to MJ/1 -> Scope1/1, MJ1/1, MJ/1, MJ to kWh/1
  MJ to kWh/1 -> Scope2/1, kWh1/1, kWh/1

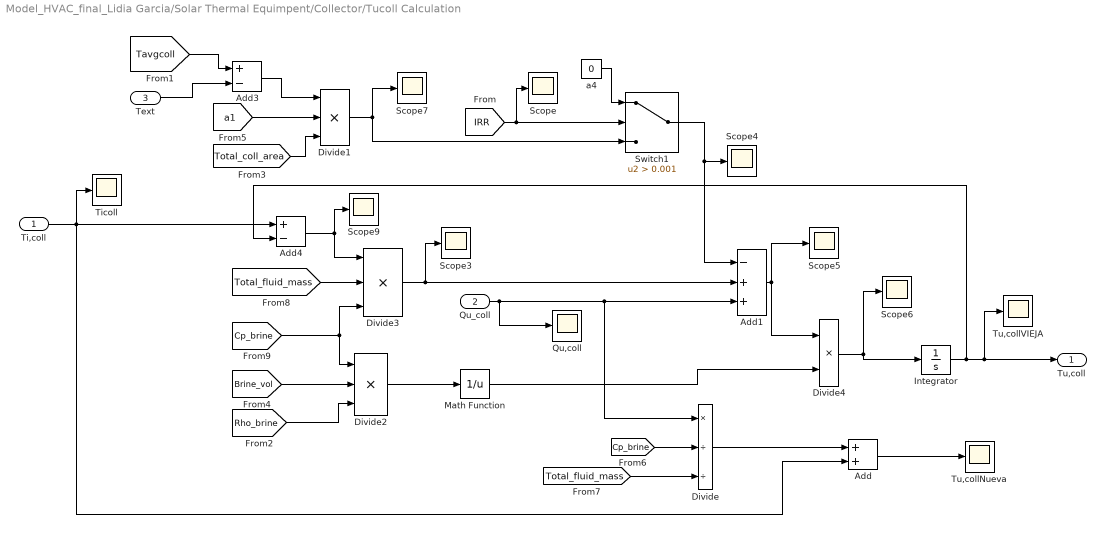
== system Model_HVAC_final_Lidia Garcia/Solar Thermal Equimpent/Collector/Tucoll Calculation ==
  Ti,coll : Inport
  Qu_coll : Inport  Port=2
  Text : Inport  Port=3
  Add : Sum
  Add1 : Sum  Inputs=-++
  Add3 : Sum  Inputs=+-
  Add4 : Sum  Inputs=+-
  Divide : Product  Inputs=*//
  Divide1 : Product  Inputs=***
  Divide2 : Product  Inputs=***
  Divide3 : Product  Inputs=***
  Divide4 : Product  Inputs=**
  Integrator : Integrator  InitialCondition=15
  Math Function : Math  Operator=reciprocal  SignedPower=on  SaturateOnIntegerOverflow=on
  Qu,coll : Scope
  Scope{,3..7,9} (7 alike) : Scope
  Switch1 : Switch  Criteria=u2 > Threshold  Threshold=0.001
  Ticoll : Scope
  Tu,collNueva : Scope
  Tu,collVIEJA : Scope
  a4 : Constant  Value=0  SampleTime=-1
  Tu,coll : Outport  VectorParamsAs1DForOutWhenUnconnected=off
  wires:
  [Tavgcoll] -> Add3/1
  Text/1 -> Add3/2
  Add3/1 -> Divide1/1
  [a1] -> Divide1/2
  Divide2/1 -> Math Function/1
  Add4/1 -> Divide3/1, Scope9/1
  Divide3/1 -> Add1/2, Scope3/1
  Qu_coll/1 -> Add1/3, Divide/1, Qu,coll/1
  Add1/1 -> Divide4/1, Scope5/1
  Math Function/1 -> Divide4/2
  Divide4/1 -> Scope6/1, Integrator/1
  Integrator/1 -> Add4/2, Tu,coll/1, Tu,collVIEJA/1
  [Total_coll_area] -> Divide1/3
  [IRR] -> Scope/1, Switch1/2
  a4/1 -> Switch1/1
  Switch1/1 -> Add1/1, Scope4/1
  Ti,coll/1 -> Ticoll/1, Add4/1, Add/2
  Divide1/1 -> Switch1/3, Scope7/1
  [Total_fluid_mass] -> Divide/3
  Add/1 -> Tu,collNueva/1
  [Cp_brine] -> Divide/2
  Divide/1 -> Add/1
  [Brine_vol] -> Divide2/2
  [Rho_brine] -> Divide2/3
  [Cp_brine] -> Divide3/3, Divide2/1
  [Total_fluid_mass] -> Divide3/2

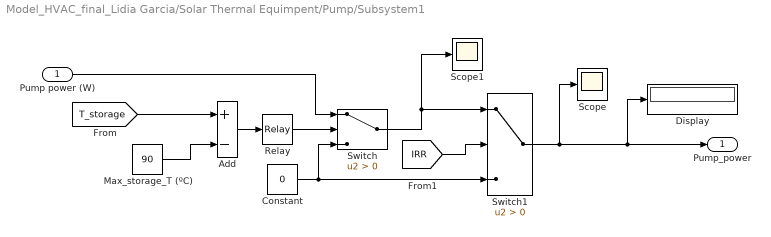
== system Model_HVAC_final_Lidia Garcia/Solar Thermal Equimpent/Pump/Subsystem1 ==
  Pump power (W) : Inport
  Add : Sum  Inputs=+-
  Constant : Constant  Value=0
  Display : Display
  Max_storage_T (ºC) : Constant  Value=90  SampleTime=-1
  Relay : Relay  OnSwitchValue=0  OffSwitchValue=-5  OnOutputValue=0  OffOutputValue=1
  Scope : Scope
  Scope1 : Scope
  Switch : Switch  Criteria=u2 > Threshold
  Switch1 : Switch  Criteria=u2 > Threshold
  Pump_power : Outport
  wires:
  Add/1 -> Relay/1
  Relay/1 -> Switch/2
  Pump power (W)/1 -> Switch/1
  Constant/1 -> Switch1/3, Switch/3
  [IRR] -> Switch1/2
  Switch/1 -> Scope1/1, Switch1/1
  Switch1/1 -> Scope/1, Pump_power/1, Display/1
  [T_storage] -> Add/1
  Max_storage_T (ºC)/1 -> Add/2

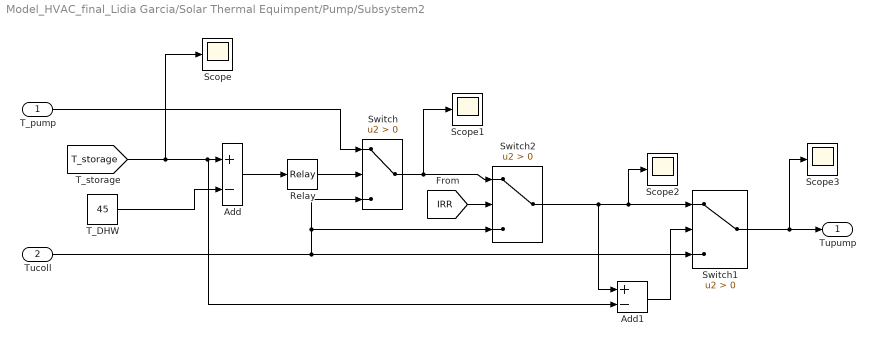
== system Model_HVAC_final_Lidia Garcia/Solar Thermal Equimpent/Pump/Subsystem2 ==
  T_pump : Inport
  Tucoll : Inport  Port=2
  Add : Sum  Inputs=+-
  Add1 : Sum  Inputs=+-
  Relay : Relay  OnSwitchValue=0  OffSwitchValue=-5  OnOutputValue=0  OffOutputValue=1
  Scope{,1..3} (4 alike) : Scope
  Switch : Switch  Criteria=u2 > Threshold
  Switch1 : Switch  Criteria=u2 > Threshold
  Switch2 : Switch  Criteria=u2 > Threshold
  T_DHW : Constant  Value=45  SampleTime=-1
  Tupump : Outport
  wires:
  [T_storage] -> Scope/1, Add1/2, Add/1
  T_DHW/1 -> Add/2
  Add/1 -> Relay/1
  Relay/1 -> Switch/2
  T_pump/1 -> Switch/1
  Tucoll/1 -> Switch/3, Switch2/3, Switch1/3
  Switch/1 -> Scope1/1, Switch2/1
  [IRR] -> Switch2/2
  Switch2/1 -> Scope2/1, Switch1/1, Add1/1
  Add1/1 -> Switch1/2
  Switch1/1 -> Scope3/1, Tupump/1

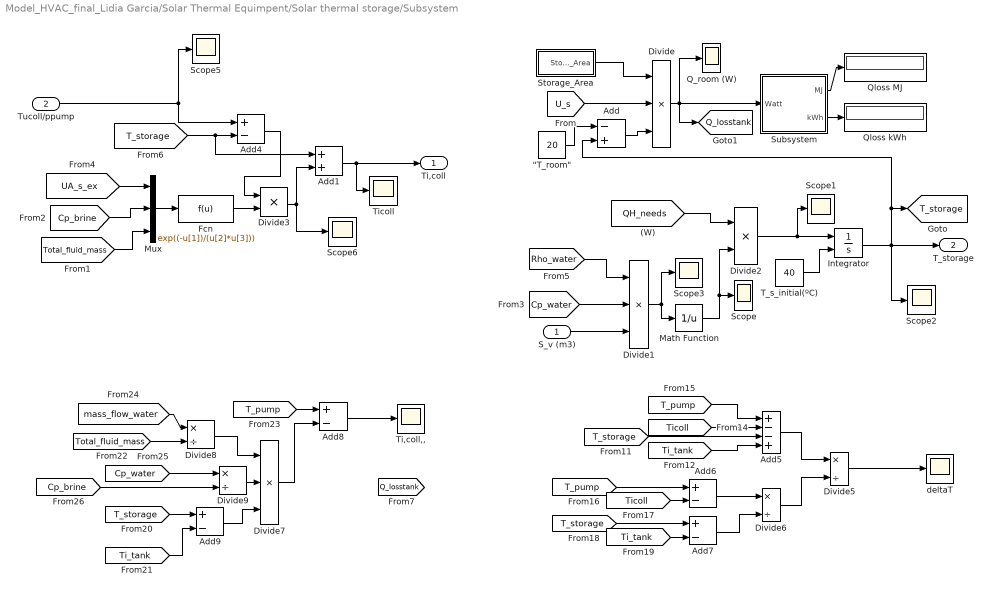
== system Model_HVAC_final_Lidia Garcia/Solar Thermal Equimpent/Solar thermal storage/Subsystem ==
  S_v (m3) : Inport
  Tucoll/ppump : Inport  Port=2
  "\"T_room\"" : Constant  Value=20
  Add : Sum  Inputs=-+
  Add1 : Sum
  Add{4,6..9} (5 alike) : Sum  Inputs=+-
  Add5 : Sum  Inputs=+--+
  Divide : Product  Inputs=***
  Divide1 : Product  Inputs=***
  Divide2 : Product  Inputs=**
  Divide3 : Product  Inputs=**
  Divide{5..6,8..9} (4 alike) : Product  Inputs=*/
  Divide7 : Product  Inputs=***
  Fcn : Fcn  Expr=exp((-u[1])/(u[2]*u[3]))
  Integrator : Integrator  InitialConditionSource=external
  Math Function : Math  Operator=reciprocal  SaturateOnIntegerOverflow=on
  Mux : Mux  Inputs=3
  Q_room (W) : Scope
  Qloss MJ : Display
  Qloss kWh : Display
  Scope{,1..3,5..6} (6 alike) : Scope
  Storage_Area : Subsystem
  Subsystem : Subsystem
  T_s_initial(ºC) : Constant  Value=40  SampleTime=-1
  Ti,coll,, : Scope
  Ticoll : Scope
  deltaT : Scope
  Ti,coll : Outport
  T_storage : Outport  Port=2
  tag scope: Q_losstank=global, T_storage=global
  wires:
  Storage_Area/1(" Storage_Area") -> Divide/1
  [U_s] -> Divide/2
  "\"T_room\""/1 -> Add/1
  Add/1 -> Divide/3
  Divide/1 -> Subsystem/1(Watt), [Q_losstank], Q_room (W)/1
  Subsystem/1(MJ) -> Qloss MJ/1
  Subsystem/2(kWh) -> Qloss kWh/1
  S_v (m3)/1 -> Divide1/3
  Math Function/1 -> Scope/1, Divide2/2
  Divide2/1 -> Integrator/1, Scope1/1
  T_s_initial(ºC)/1 -> Integrator/2
  Integrator/1 -> T_storage/1, [T_storage], Add/2, Scope2/1
  Divide1/1 -> Math Function/1, Scope3/1
  [QH_needs] -> Divide2/1
  [Cp_water] -> Divide1/2
  [Rho_water] -> Divide1/1
  [Cp_brine] -> Mux/2
  Divide3/1 -> Scope6/1, Add1/2
  [UA_s_ex] -> Mux/1
  Tucoll/ppump/1 -> Add4/1, Scope5/1
  [T_storage] -> Add1/1, Add4/2
  Fcn/1 -> Divide3/2
  Mux/1 -> Fcn/1
  Add4/1 -> Divide3/1
  [Total_fluid_mass] -> Mux/3
  Add1/1 -> Ticoll/1, Ti,coll/1
  Add5/1 -> Divide5/1
  Divide6/1 -> Divide5/2
  Add7/1 -> Divide6/2
  Add6/1 -> Divide6/1
  [T_pump] -> Add5/1
  [Ticoll] -> Add5/2
  [T_storage] -> Add5/3
  [Ti_tank] -> Add5/4
  [T_pump] -> Add6/1
  [Ticoll] -> Add6/2
  [T_storage] -> Add7/1
  [Ti_tank] -> Add7/2
  Divide5/1 -> deltaT/1
  [T_pump] -> Add8/1
  Divide8/1 -> Divide7/1
  Divide9/1 -> Divide7/2
  Add9/1 -> Divide7/3
  [mass_flow_water] -> Divide8/1
  [Total_fluid_mass] -> Divide8/2
  [Cp_water] -> Divide9/1
  [Cp_brine] -> Divide9/2
  [T_storage] -> Add9/1
  [Ti_tank] -> Add9/2
  Divide7/1 -> Add8/2
  Add8/1 -> Ti,coll,,/1

== system Model_HVAC_final_Lidia Garcia/Solar Thermal Equimpent/Solar thermal storage/Subsystem/Storage_Area ==
  Add : Sum
  Constant4 : Constant  Value=2
  Display : Display
  Divide : Product  Inputs=***
  Divide1 : Product  Inputs=****
  Gain : Gain  Gain=0.5
  Math Function : Math  Operator=square  SaturateOnIntegerOverflow=on
  pi : Constant  Value=3.14
  " Storage_Area" : Outport
  wires:
  Add/1 -> " Storage_Area"/1, Display/1
  Math Function/1 -> Divide/3
  Gain/1 -> Divide1/4, Math Function/1
  [D_s] -> Gain/1
  Constant4/1 -> Divide/1, Divide1/2
  pi/1 -> Divide/2, Divide1/3
  [H_s] -> Divide1/1
  Divide/1 -> Add/1
  Divide1/1 -> Add/2

== system Model_HVAC_final_Lidia Garcia/Solar Thermal Equimpent/Solar thermal storage/Subsystem/Subsystem ==
  Watt : Inport
  Display : Display
  Display1 : Display
  Integrator : Integrator
  J to MJ : Gain  Gain=1/1000000
  MJ to kWh : Gain  Gain=1/3.6
  Scope : Scope
  Scope1 : Scope
  MJ : Outport
  kWh : Outport  Port=2
  wires:
  Watt/1 -> Integrator/1
  Integrator/1 -> J to MJ/1
  J to MJ/1 -> MJ/1, Display/1, Scope/1, MJ to kWh/1
  MJ to kWh/1 -> kWh/1, Display1/1, Scope1/1
